simulink model "Q1_model"  (R2020b)
settings: Solver=VariableStepAuto  StartTime=0.0  StopTime=400  RelTol=1e-3
model workspace (MATLAB code in the model file):
  | Ti = 549.67;
  | Cp = 0.8;
  | pho = 52;
  | delta_Hr = -500*10^3;
  | V = 1200;
  | Fi = 20;
  | alpha = 2.4*10^15;
  | beta = 2*10^4;
  | Cp = 1.05506*10^3*0.8; % Converted to kJ/lb
  | CAiss = 0.8;
  | Tinit = 559;
  | CAinit = 0.0193;
settings Model: Creator=HP  LastModifiedBy=HP

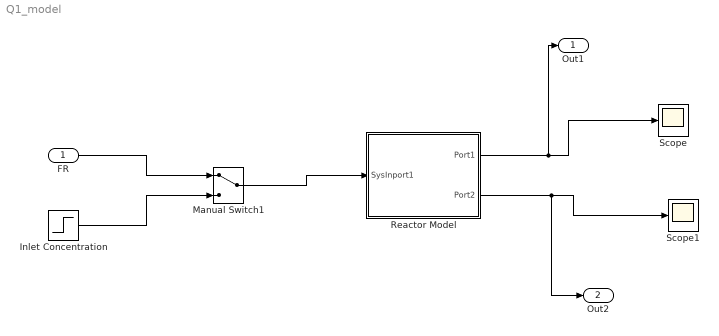
== system Q1_model ==
  FR : Inport
  Inlet Concentration : Step  Time=0  Before=CAiss  After=CAiss*1.1  SampleTime=0
  Manual Switch1 : ManualSwitch
  Reactor Model : Subsystem  mask(Differential Equation Editor (DEE)){}
      settings: OpenFcn=diffeqed
      mask Display: disp('Reactor')
  Scope : Scope
  Scope1 : Scope
  Out1 : Outport  SignalName=Concentration
  Out2 : Outport  Port=2  SignalName=Temperature
  wires:
  Reactor Model/1(Port1) -> Out1/1, Scope/1
  Reactor Model/2(Port2) -> Out2/1, Scope1/1
  Manual Switch1/1 -> Reactor Model/1(SysInport1)
  FR/1 -> Manual Switch1/1
  Inlet Concentration/1 -> Manual Switch1/2

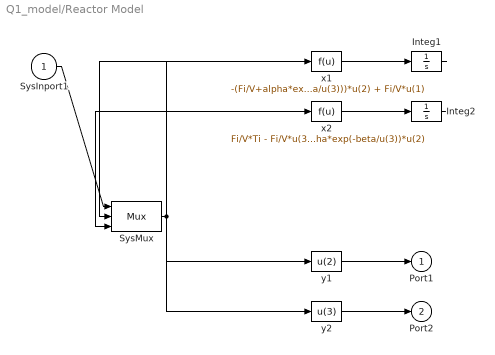
== system Q1_model/Reactor Model ==
  SysInport1 : Inport
  Integ1 : Integrator  InitialCondition=CAinit
  Integ2 : Integrator  InitialCondition=Tinit
  SysMux : Mux  Inputs=3
  x1 : Fcn  Expr=-(Fi/V+alpha*exp(-beta/u(3)))*u(2) + Fi/V*u(1)
  x2 : Fcn  Expr=Fi/V*Ti - Fi/V*u(3) - (delta_Hr)/(pho*Cp)*alpha*exp(-beta/u(3))*u(2)
  y1 : Fcn  Expr=u(2)
  y2 : Fcn  Expr=u(3)
  Port1 : Outport  InitialOutput=0
  Port2 : Outport  Port=2
  wires:
  SysInport1/1 -> SysMux/1
  SysMux/1 -> x1/1, x2/1, y1/1, y2/1
  x1/1 -> Integ1/1
  Integ1/1 -> SysMux/2
  x2/1 -> Integ2/1
  Integ2/1 -> SysMux/3
  y1/1 -> Port1/1
  y2/1 -> Port2/1
